simulink model "expt6_2"  (R2019a)
settings: Solver=VariableStepAuto  StartTime=0.0  StopTime=0.1  RelTol=1e-3
libraries: simulink_extras x8, dspsigops x2, commsrccod2 x2, commutil2 x1, simulink x1, dspquant2 x1, dsparch4 x1
settings Model: Creator=hp  LastModifiedBy=hp

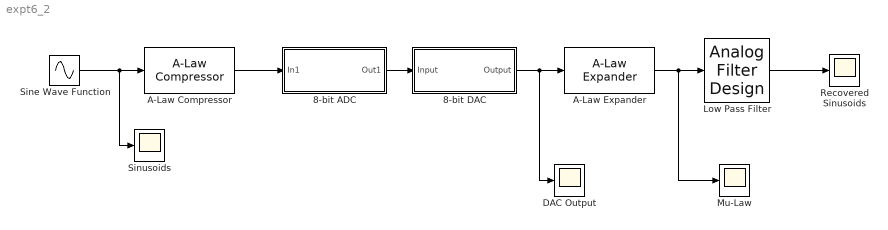
== system expt6_2 ==
  8-bit ADC : Subsystem
  8-bit DAC : Subsystem
  A-Law Compressor : commsrccod2/A-Law Compressor  A=87.6  V=1
      settings: SourceProductName=Communications Toolbox  SourceProductBaseCode=CM
  A-Law Expander : commsrccod2/A-Law Expander  A=87.6  V=1
      settings: SourceProductName=Communications Toolbox  SourceProductBaseCode=CM
  DAC Output : Scope
  Low Pass Filter : dsparch4/Analog Filter Design  method=Butterworth  filttype=Lowpass  N=8  Wlo=2*pi*350  Whi=80  Rp=2  Rs=40
  Mu-Law : Scope
  Recovered Sinusoids : Scope
  Sine Wave Function : Sin  Frequency=2*pi*300  SampleTime=0
  "Sinusoids " : Scope
  wires:
  8-bit DAC/1(Output) -> DAC Output/1, A-Law Expander/1
  8-bit ADC/1(Out1) -> 8-bit DAC/1(Input)
  A-Law Compressor/1 -> 8-bit ADC/1(In1)
  Sine Wave Function/1 -> "Sinusoids "/1, A-Law Compressor/1
  A-Law Expander/1 -> Low Pass Filter/1, Mu-Law/1
  Low Pass Filter/1 -> Recovered Sinusoids/1

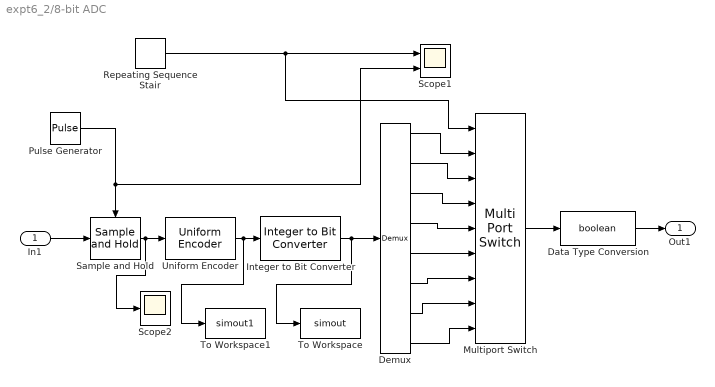
== system expt6_2/8-bit ADC ==
  In1 : Inport
  Data Type Conversion : DataTypeConversion  OutDataTypeStr=boolean
  Demux : Demux  Outputs=8
  Integer to Bit Converter : commutil2/Integer to Bit Converter  nbits=8  signedInputValues=Unsigned  bitOrder=MSB first  outDtype=Inherit via internal rule
      settings: SourceProductName=Communications Toolbox
  Multiport Switch : MultiPortSwitch  Inputs=8
  Pulse Generator : DiscretePulseGenerator  PulseType=Time based  Period=1/8000  PulseWidth=50
  Repeating Sequence Stair : simulink/Sources/Repeating Sequence Stair  OutValues=[1 2 3 4 5 6 7 8].'  tsamp=1/64000  OutMin=[]  OutMax=[]  OutDataTypeStr=double  OutputDataTypeScalingMode=double  OutDataType=fixdt(0,8)  ConRadixGroup=Best Precision: Vector-wise  OutScaling=2^-12
  Sample and Hold : dspsigops/Sample and Hold  trig=Rising edge  initCond=0  latchinput=off
  Scope1 : Scope  NumInputPorts=2
  Scope2 : Scope
  To Workspace : ToWorkspace  VariableName=simout  SaveFormat=Timeseries  SampleTime=-1
  To Workspace1 : ToWorkspace  VariableName=simout1  SaveFormat=Timeseries  SampleTime=-1
  Uniform Encoder : dspquant2/Uniform Encoder  peak=1.3  bits=8  otype=Unsigned integer
      settings: SourceProductName=DSP System Toolbox
  Out1 : Outport
  wires:
  In1/1 -> Sample and Hold/1
  Uniform Encoder/1 -> To Workspace1/1, Integer to Bit Converter/1
  Integer to Bit Converter/1 -> To Workspace/1, Demux/1
  Demux/8 -> Multiport Switch/9
  Demux/7 -> Multiport Switch/8
  Demux/6 -> Multiport Switch/7
  Demux/5 -> Multiport Switch/6
  Demux/4 -> Multiport Switch/5
  Demux/3 -> Multiport Switch/4
  Demux/2 -> Multiport Switch/3
  Demux/1 -> Multiport Switch/2
  Sample and Hold/1 -> Scope2/1, Uniform Encoder/1
  Repeating Sequence Stair/1 -> Scope1/1, Multiport Switch/1
  Pulse Generator/1 -> Scope1/2, Sample and Hold/Trigger
  Multiport Switch/1 -> Data Type Conversion/1
  Data Type Conversion/1 -> Out1/1

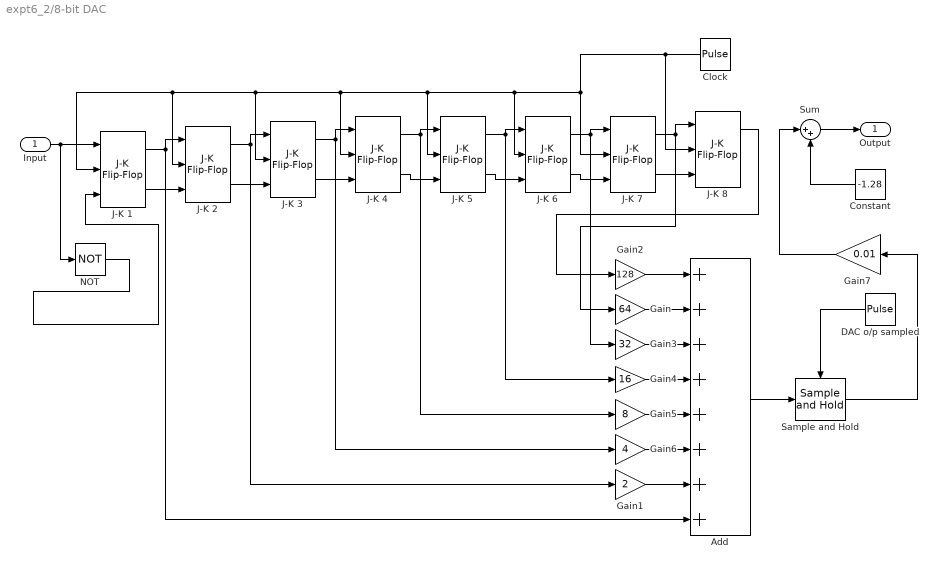
== system expt6_2/8-bit DAC ==
  Input : Inport
  Add : Sum  Inputs=8
  Clock : DiscretePulseGenerator  PulseType=Time based  Period=1/64000  PulseWidth=50
  Constant : Constant  Value=-1.28
  DAC o/p sampled : DiscretePulseGenerator  PulseType=Time based  Period=1/8000  PulseWidth=50
  Gain : Gain  Gain=64
  Gain1 : Gain  Gain=2
  Gain2 : Gain  Gain=128
  Gain3 : Gain  Gain=32
  Gain4 : Gain  Gain=16
  Gain5 : Gain  Gain=8
  Gain6 : Gain  Gain=4
  Gain7 : Gain  Gain=0.01
  J-K {1..8} (8 alike) : simulink_extras/Flip Flops/J-K Flip-Flop  initial_condition=0
      settings: SourceProductName=Simulink
  NOT : Logic  Operator=NOT  IconShape=distinctive  AllPortsSameDT=off  OutDataTypeStr=boolean
  Sample and Hold : dspsigops/Sample and Hold  trig=Rising edge  initCond=0  latchinput=off
  Sum : Sum  Inputs=|++
  Output : Outport
  wires:
  Input/1 -> NOT/1, J-K 1/1
  Constant/1 -> Sum/2
  Add/1 -> Sample and Hold/1
  DAC o/p sampled/1 -> Sample and Hold/Trigger
  Sample and Hold/1 -> Gain7/1
  Gain2/1 -> Add/1
  Gain/1 -> Add/2
  Gain3/1 -> Add/3
  Gain4/1 -> Add/4
  Gain5/1 -> Add/5
  Gain6/1 -> Add/6
  Gain1/1 -> Add/7
  J-K 1/1 -> J-K 2/1, Add/8
  J-K 2/1 -> J-K 3/1, Gain1/1
  J-K 3/1 -> J-K 4/1, Gain6/1
  J-K 4/1 -> J-K 5/1, Gain5/1
  J-K 5/1 -> J-K 6/1, Gain4/1
  J-K 6/1 -> J-K 7/1, Gain3/1
  J-K 7/1 -> J-K 8/1, Gain/1
  J-K 8/1 -> Gain2/1
  Sum/1 -> Output/1
  J-K 7/2 -> J-K 8/3
  J-K 6/2 -> J-K 7/3
  J-K 5/2 -> J-K 6/3
  J-K 4/2 -> J-K 5/3
  J-K 3/2 -> J-K 4/3
  J-K 1/2 -> J-K 2/3
  Clock/1 -> J-K 8/2, J-K 7/2, J-K 6/2, J-K 5/2, J-K 4/2, J-K 3/2, J-K 2/2, J-K 1/2
  NOT/1 -> J-K 1/3
  Gain7/1 -> Sum/1
  J-K 2/2 -> J-K 3/3
